simulink model "ECB"  (R2017a)
settings: Solver=ode4  StartTime=0.0  StopTime=1548.3  FixedStep=0.001  RelTol=1e-3  EnableMultiTasking=on
undefined symbols (not defined in the file or in its folder): magnitude, sgn, sigbuilder_block
libraries: simulink x1
(part 2 of 2)

== system ECB/ECB Model/Driver, Ctrl & Motor/AC-motor/Voltage Equations ==
  us : Inport
  is : Inport  Port=2
  wM : Inport  Port=3
  Gain1 : Gain  Gain=1i*p
  Gain2 : Gain  Gain=Rs
  Integrator (Complex Signal) : Subsystem
      mask Display: disp('1/s');
  Product : Product
  Sum1 : Sum  Inputs=+--
  psis : Outport
  wires:
  wM/1 -> Gain1/1
  Integrator (Complex Signal)/1(y) -> psis/1, Product/2
  Sum1/1 -> Integrator (Complex Signal)/1(u)
  us/1 -> Sum1/1
  Gain1/1 -> Product/1
  Product/1 -> Sum1/3
  is/1 -> Gain2/1
  Gain2/1 -> Sum1/2

== system ECB/ECB Model/Driver, Ctrl & Motor/Driver/Cycle ==
  Demux : Demux  Tag=STV Demux  Outputs=1
  FromWs : FromWorkspace  Tag=STV FromWs  VariableName=tuvar  SampleTime=0  OutputAfterFinalValue=Setting to zero
      SigBuilderData=|
      | common.afterFinalStr = 'Set to zero'
      | common.sampleTime = '0'
      | dataSet(1).timeRange = [0 1548.3]
      | dataSet(1).name = 'E11_TFBest'
      | dataSet(2).timeRange = [0 1767.7]
      | dataSet(2).name = 'Brauschweig'
      | dataSet(3).timeRange = [0 1548.3]
      | dataSet(3).name = 'NYbus'
      | dataSet(4).timeRange = [0 1698.1]
      | dataSet(4).name = 'ft5v'
      | dataSet(5).timeRange = [0 1548.3]
      | dataSet(5).name = 'ft9v'
      | dataSet(6).timeRange = [0 1548.3]
      | dataSet(6).name = 'ft11v'
      | dataSet(7).timeRange = [0 1549.6]
      | dataSet(7).name = 'ft19v'
      | dataSet(8).timeRange = [0 1798.1]
      | dataSet(8).name = 'ft25v'
      | dataSet(9).timeRange = [0 2058.9]
      | dataSet(9).name = 'tf4v'
      | dataSet(10).timeRange = [0 1565.4]
      | dataSet(10).name = 'tf8v'
      | dataSet(11).timeRange = [0 1548.3]
      | dataSet(11).name = 'tf12v'
      | dataSet(12).timeRange = [0 1569]
      | dataSet(12).name = 'tf22v'
      | dataSet(13).timeRange = [0 1548.3]
      | dataSet(13).name = 'tf24v'
      | sbobj.Name = 'Signal Builder'
      | sbobj.Groups(1).Name = 'E11_TFBest'
      | sbobj.Groups(1).Signals.Name = 'vel'
      | sbobj.Groups(1).Signals.XData = [0 0.1 0.2 0.3 0.4 0.5 0.6 0.7 0.8 0.9 1 1.1 ... (15484 elements, 1x15484)]
      | sbobj.Groups(1).Signals.YData = [0 0 0 0 0 0 0 0 0 0 0 0 ... (15484 elements, 1x15484)]
      | sbobj.Groups(1).TimeRange = [0 1548.3]
      | sbobj.Groups(2).Name = 'Brauschweig'
      | sbobj.Groups(2).Signals.Name = 'vel'
      | sbobj.Groups(2).Signals.XData = [0 0.09 0.2 0.3 0.39 0.5 0.59 0.7 0.8 0.89 1 1.09 ... (17678 elements, 1x17678)]
      | sbobj.Groups(2).Signals.YData = [1.0444e-14 1.3228e-14 1.6325e-14 1.9741e-14 2.3481e-14 2.7541e-14 3.1914e-14 3.6586e-14 4.1533e-14 4.6723e-14 5.2115e-14 5.7653e-14 ... (17678 elements, 1x17678)]
      | sbobj.Groups(2).TimeRange = [0 1767.7]
      | sbobj.Groups(3).Name = 'NYbus'
      | sbobj.Groups(3).Signals.Name = 'vel'
      | sbobj.Groups(3).Signals.XData = [0 14.4398340249 15.569428651 16.6194998155 17.1824897772 18.2271388874 20.195344564 22.1671649434 24.6947458789 24.7290855555 25.2468917321 27.1554548124 27.5377096339 27.9922585115 29.4571168227 29.9134730516 31.3692946058 59.7510373444 60.2814949808 61.438199878 62.5714092069 62.6418959116 63.6666641565 64.6769735901 67.1159943068 70.1631887703 73.0892906899 75.1352124767 76.7844206309 78.4209773253 78.9839672869 79.0255363692 80.5446152224 82.9800212364 84.4231913307 86.488993983 88.8864456175 89.7991580755 91.1555753025 92.4794602044 94.3609130137 95.6956420239 97.5933609959 163.815620034 165.336506239 165.977212311 168.109886965 171.063099156 171.887251395 174.273858921 209.128630705 211.228773034 212.935816433 214.5 216.99332033 220.020633929 221.936426414 223.32899067 225.194177316 225.243571477 226.617466545 227.55186722 232.033195021 233.595650308 234.147796161 234.758311934 235.304501058 236.762129964 237.184146516 240.133744004 243.240581063 246.154031523 247.063129278 248.962655602 284.813278008 287.056201098 288.723482766 291.678502308 294.718467366 297.409613603 300.248962656 330.124481328 331.808029159 332.961119353 334.067218411 337.485823587 340.536632754 343.935357065 344.822766603 346.208101453 346.637347411 350.041493776 389.377593361 391.017764758 391.618709099 394.157134143 398.586048753 400.641007297 402.192618476 404.065034528 405.416029701 407.302904564 434.68879668 435.789473684 436.910031553 438.4851383 441.858559692 442.242621864 445.147035567 479.502074689 481.133209329 482.298950983 484.368368338 486.332959312 488.402376667 491.85532152 494.991076202 496.96108923 499.486862814 502.907275342 504.269114624 506.108998351 507.470837632 510.373443983 555.186721992 556.347041592 557.932992447 557.983598286 562.425164356 565.506698496 568.311707872 569.697042721 572.614107884 1548.3]
      | sbobj.Groups(3).Signals.YData = [0 0 7.56479303085 10.6316010163 14.3117705989 17.0718977858 15.7429476588 14.6184513975 16.7652169873 18.7075287114 19.8320249728 15.1295860617 8.58706235935 6.13361597096 4.49798504537 2.14676558984 0 0 1.84008479129 10.9382818149 18.7075287114 22.6943790926 24.3300100181 25.1478254809 22.2854713612 25.6589601452 22.1832444283 25.2500524138 34.0415686388 42.1174963339 45.7976659165 48.1488853721 49.5800624319 46.5132544465 43.6509003267 47.8422045735 42.6286309982 37.9261920871 30.1569451906 20.5476135027 14.3117705989 5.31580050817 0 0 1.43117705989 9.50710475499 17.4808055172 15.5384937931 5.82693517241 0 0 6.13361597096 18.1963940472 23.5 22.387698294 24.6366908167 20.343159637 14.6184513975 7.462566098 4.60021197822 3.47571571688 0 0 3.88462344828 6.95143143376 13.0850474047 16.0496284574 14.0050898004 9.71155862069 7.56479303085 14.3117705989 10.1204663521 5.21357357532 0 0 14.2095436661 24.0233292196 22.1832444283 25.1478254809 8.38260849365 0 0 10.7338279492 19.6275711071 25.8634140109 22.0810174955 25.6589601452 20.7520673684 14.6184513975 8.4848354265 4.60021197822 0 0 8.2803815608 14.1073167332 16.8674439201 13.9028628675 17.4808055172 20.7520673684 14.0050898004 5.92916210526 0 0 5.92916210526 12.9828204719 17.5830324501 11.2449626134 4.80466584392 0 0 7.76924689655 17.3785785844 21.7743366969 20.2409327042 24.6366908167 22.7966060254 31.1792145191 29.9524913249 31.9970299819 28.3168603993 20.8542943013 12.2672319419 4.80466584392 0 0 9.30265088929 14.5162244646 17.3785785844 15.1295860617 20.4453865699 10.1204663521 3.98685038113 0 0]
      | sbobj.Groups(3).TimeRange = [0 1548.3]
      | sbobj.Groups(4).Name = 'ft5v'
      | sbobj.Groups(4).Signals.Name = 'vel'
      | sbobj.Groups(4).Signals.XData = [0 0.1 0.2 0.3 0.4 0.5 0.6 0.7 0.8 0.9 1 1.1 ... (16982 elements, 1x16982)]
      | sbobj.Groups(4).Signals.YData = [3.68548 3.78425333333 3.859568 4.08498285714 4.35425777778 4.58117454545 4.78955692308 5.01645066667 5.233752 5.448584 5.66218133333 5.922696 ... (16982 elements, 1x16982)]
      | sbobj.Groups(4).TimeRange = [0 1698.1]
      | sbobj.Groups(5).Name = 'ft9v'
      | sbobj.Groups(5).Signals.Name = 'vel'
      | sbobj.Groups(5).Signals.XData = [0 0.1 0.2 0.3 0.4 0.5 0.6 0.7 0.8 0.9 1 1.1 ... (14571 elements, 1x14571)]
      | sbobj.Groups(5).Signals.YData = [4.57444 4.92014666667 5.318944 5.75442857143 6.18568 6.59480363636 7.04329846154 7.48701866667 7.90557066667 8.34017333333 8.75996 9.17974666667 ... (14571 elements, 1x14571)]
      | sbobj.Groups(5).TimeRange = [0 1548.3]
      | sbobj.Groups(6).Name = 'ft11v'
      | sbobj.Groups(6).Signals.Name = 'vel'
      | sbobj.Groups(6).Signals.XData = [0 0.1 0.2 0.3 0.4 0.5 0.6 0.7 0.8 0.9 1 1.1 ... (13984 elements, 1x13984)]
      | sbobj.Groups(6).Signals.YData = [1.27788 1.33344 1.46308 1.53980571429 1.66268444444 1.76613454545 1.87906769231 1.99892533333 2.11004533333 2.21005333333 2.31746933333 2.42118133333 ... (13984 elements, 1x13984)]
      | sbobj.Groups(6).TimeRange = [0 1548.3]
      | sbobj.Groups(7).Name = 'ft19v'
      | sbobj.Groups(7).Signals.Name = 'vel'
      | sbobj.Groups(7).Signals.XData = [0 0.1 0.2 0.3 0.4 0.5 0.6 0.7 0.8 0.9 1 1.1 ... (15497 elements, 1x15497)]
      | sbobj.Groups(7).Signals.YData = [3.8892 4.21021333333 4.544808 4.92102857143 5.34610666667 5.71931272727 6.08168307692 6.378288 6.69806666667 6.993152 7.29194133333 7.58826133333 ... (15497 elements, 1x15497)]
      | sbobj.Groups(7).TimeRange = [0 1549.6]
      | sbobj.Groups(8).Name = 'ft25v'
      | sbobj.Groups(8).Signals.Name = 'vel'
      | sbobj.Groups(8).Signals.XData = [0 0.1 0.2 0.3 0.4 0.5 0.6 0.7 0.8 0.9 1 1.1 ... (17982 elements, 1x17982)]
      | sbobj.Groups(8).Signals.YData = [4.92632 5.43870666667 5.752312 6.23330285714 6.68777777778 7.04433454545 7.40515076923 7.752472 8.10682133333 8.42166133333 8.71304266667 9.02417866667 ... (17982 elements, 1x17982)]
      | sbobj.Groups(8).TimeRange = [0 1798.1]
      | sbobj.Groups(9).Name = 'tf4v'
      | sbobj.Groups(9).Signals.Name = 'vel'
      | sbobj.Groups(9).Signals.XData = [0 0.1 0.2 0.3 0.4 0.5 0.6 0.7 0.8 0.9 1 1.1 ... (20590 elements, 1x20590)]
      | sbobj.Groups(9).Signals.YData = [2.53724 2.86442666667 3.174328 3.52144571429 3.72252 3.88751636364 4.10146769231 4.374424 4.64605066667 4.90533066667 5.17201866667 5.45352266667 ... (20590 elements, 1x20590)]
      | sbobj.Groups(9).TimeRange = [0 2058.9]
      | sbobj.Groups(10).Name = 'tf8v'
      | sbobj.Groups(10).Signals.Name = 'vel'
      | sbobj.Groups(10).Signals.XData = [0 0.1 0.2 0.3 0.4 0.5 0.6 0.7 0.8 0.9 1 1.1 ... (15655 elements, 1x15655)]
      | sbobj.Groups(10).Signals.YData = [0 0 0 0 0 0 0 0 0 0 0 0 ... (15655 elements, 1x15655)]
      | sbobj.Groups(10).TimeRange = [0 1565.4]
      | sbobj.Groups(11).Name = 'tf12v'
      | sbobj.Groups(11).Signals.Name = 'vel'
      | sbobj.Groups(11).Signals.XData = [0 0.1 0.2 0.3 0.4 0.5 0.6 0.7 0.8 0.9 1 1.1 ... (14670 elements, 1x14670)]
      | sbobj.Groups(11).Signals.YData = [5.05596 5.07448 5.193008 5.51896 5.82145333333 6.13517090909 6.42216615385 6.73881066667 7.026488 7.33638933333 7.66110666667 7.99446666667 ... (14670 elements, 1x14670)]
      | sbobj.Groups(11).TimeRange = [0 1548.3]
      | sbobj.Groups(12).Name = 'tf22v'
      | sbobj.Groups(12).Signals.Name = 'vel'
      | sbobj.Groups(12).Signals.XData = [0 0.1 0.2 0.3 0.4 0.5 0.6 0.7 0.8 0.9 1 1.1 ... (15691 elements, 1x15691)]
      | sbobj.Groups(12).Signals.YData = [15.53828 14.3962133333 14.22336 14.1783828571 14.4414844444 14.6038618182 14.8444923077 15.0962693333 15.182696 15.4185173333 15.664216 15.9259653333 ... (15691 elements, 1x15691)]
      | sbobj.Groups(12).TimeRange = [0 1569]
      | sbobj.Groups(13).Name = 'tf24v'
      | sbobj.Groups(13).Signals.Name = 'vel'
      | sbobj.Groups(13).Signals.XData = [0 0.1 0.2 0.3 0.4 0.5 0.6 0.7 0.8 0.9 1 1.1 ... (15122 elements, 1x15122)]
      | sbobj.Groups(13).Signals.YData = [2.4076 2.48168 2.489088 2.51342857143 2.58868444444 2.69718545455 2.81361538462 2.92739466667 3.03481066667 3.144696 3.241 3.366936 ... (15122 elements, 1x15122)]
      | sbobj.Groups(13).TimeRange = [0 1548.3]
  vel : Outport  Tag=STV Outport
  wires:
  Demux/1 -> vel/1
  FromWs/1 -> Demux/1

== system ECB/ECB Model/Driver, Ctrl & Motor/Driver/Signal Builder ==
  Demux : Demux  Tag=STV Demux  Outputs=1
  FromWs : FromWorkspace  Tag=STV FromWs  VariableName=tuvar  SampleTime=0
      SigBuilderData=|
      | common.afterFinalStr = 'Extrapolate'
      | common.sampleTime = 0
      | dataSet.timeRange = [0 60]
      | dataSet.name = 'Group 1'
      | sbobj.Groups.Name = 'Group 1'
      | sbobj.Groups.Signals.Name = 'Signal 1'
      | sbobj.Groups.Signals.XData = [0 5 20 35 55 60]
      | sbobj.Groups.Signals.YData = [0 0 60 60 0 0]
      | sbobj.Groups.TimeRange = [0 60]
  Signal 1 : Outport  Tag=STV Outport
  wires:
  Demux/1 -> Signal 1/1
  FromWs/1 -> Demux/1

== system ECB/ECB Model/Driver, Ctrl & Motor/PID Current Ctrl/Derivative (Complex Signla) ==
  x : Inport
  Complex to Real-Imag : ComplexToRealImag
  Derivative : Derivative
  Derivative1 : Derivative
  Real-Imag to Complex : RealImagToComplex
  dx : Outport
  wires:
  Complex to Real-Imag/2 -> Derivative1/1
  Real-Imag to Complex/1 -> dx/1
  Derivative1/1 -> Real-Imag to Complex/2
  x/1 -> Complex to Real-Imag/1
  Derivative/1 -> Real-Imag to Complex/1
  Complex to Real-Imag/1 -> Derivative/1

== system ECB/ECB Model/Driver, Ctrl & Motor/PID Current Ctrl/Integrator (Complex Signal) ==
  u : Inport
  Complex to Real-Imag : ComplexToRealImag
  Integrator : Integrator
  Integrator1 : Integrator
  Real-Imag to Complex : RealImagToComplex
  y : Outport
  wires:
  u/1 -> Complex to Real-Imag/1
  Real-Imag to Complex/1 -> y/1
  Integrator1/1 -> Real-Imag to Complex/2
  Integrator/1 -> Real-Imag to Complex/1
  Complex to Real-Imag/2 -> Integrator1/1
  Complex to Real-Imag/1 -> Integrator/1

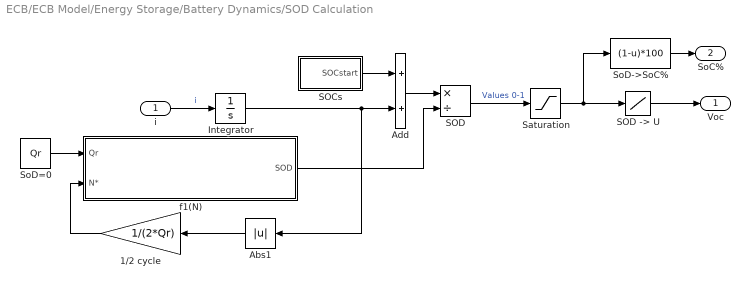
== system ECB/ECB Model/Energy Storage/Battery Dynamics/SOD Calculation ==
  i : Inport
  1/2 cycle : Gain  Gain=1/(2*Qr)
  Abs1 : Abs
  Add : Sum
  Integrator : Integrator
  SOCs : Subsystem
  SOD : Product  Inputs=*/
  "SOD -> U" : Lookup_n-D  NumberOfTableDimensions=1  BreakpointsForDimension1=SOD  BreakpointsForDimension2=[4.2,2.5]  BreakpointsForDimension3=[5, 7]  Table=VOLT  InternalRulePriority=Speed  RndMeth=Simplest  InputSameDT=on
  Saturation : Saturate  UpperLimit=1  LowerLimit=0
  SoD->SoC% : Fcn  Expr=(1-u)*100
  SoD=0 : Constant  Value=Qr
  f1(N) : Subsystem
  Voc : Outport
  SoC% : Outport  Port=2
  wires:
  SOD/1 -> Saturation/1  "Values 0-1"
  SoD=0/1 -> f1(N)/1(Qr)
  1/2 cycle/1 -> f1(N)/2(N*)
  "SOD -> U"/1 -> Voc/1
  Abs1/1 -> 1/2 cycle/1
  Add/1 -> SOD/1
  i/1 -> Integrator/1  "i"
  SoD->SoC%/1 -> SoC%/1
  f1(N)/1(SOD) -> SOD/2
  Saturation/1 -> SoD->SoC%/1, "SOD -> U"/1
  SOCs/1(SOCstart) -> Add/1
  Integrator/1 -> Add/2, Abs1/1

== system ECB/ECB Model/Driver, Ctrl & Motor/AC-motor/Voltage Equations/Integrator (Complex Signal) ==
  u : Inport
  Complex to Real-Imag : ComplexToRealImag
  Integrator : Integrator
  Integrator1 : Integrator
  Real-Imag to Complex : RealImagToComplex
  y : Outport
  wires:
  u/1 -> Complex to Real-Imag/1
  Real-Imag to Complex/1 -> y/1
  Integrator1/1 -> Real-Imag to Complex/2
  Integrator/1 -> Real-Imag to Complex/1
  Complex to Real-Imag/2 -> Integrator1/1
  Complex to Real-Imag/1 -> Integrator/1

== system ECB/ECB Model/Energy Storage/Battery Dynamics/SOD Calculation/SOCs ==
  SOC0 : Gain  Gain=1-(SOC0/100)
  Soc=? : Constant  Value=Qr
  SOCstart : Outport
  wires:
  SOC0/1 -> SOCstart/1
  Soc=?/1 -> SOC0/1

== system ECB/ECB Model/Energy Storage/Battery Dynamics/SOD Calculation/f1(N) ==
  Qr : Inport
  N* : Inport  Port=2
  N+N* : Sum
  N+N*1 : Sum  Inputs=+-
  N0 : Constant  Value=N0
  Product1 : Product
  f1(N)1 : Gain  Gain=0.2/Nnom
  SOD : Outport
  wires:
  Qr/1 -> N+N*1/1, f1(N)1/1
  Product1/1 -> N+N*1/2
  f1(N)1/1 -> Product1/1
  N+N*/1 -> Product1/2
  N0/1 -> N+N*/1
  N*/1 -> N+N*/2
  N+N*1/1 -> SOD/1

== matlab function ECB/ECB Model/Driver, Ctrl & Motor/PID Current Ctrl/MATLAB Function ==
  data: usref input; usref_saturated output; Umax input; usref_limit output
function [usref_saturated, usref_limit] = fcn(usref, Umax)
%#codegen

im1 = imag(usref);
re1 = real(usref);
alpha = atan2(im1,re1);

uref = sqrt(im1^2+re1^2);

if uref > (2/3)*Umax
    
    im2 = (2/3)*Umax*sin(alpha);
    re2 = (2/3)*Umax*cos(alpha);
    usref_saturated = re2+1i*im2;
    
else
    
    usref_saturated = usref;
    
end

usref_limit = sqrt(((2/3)*Umax*sin(alpha))^2+((2/3)*Umax*cos(alpha))^2);

== matlab function ECB/ECB Model/Driver, Ctrl & Motor/Regenerative Braking and Current Limits/MATLAB Function ==
  data: isref input; is_limited output; Ich_m input; soc input; brakes output; Ids_max output; Ich_max output; soclim input; v input; vlimPartial input; a input; alimPartial input; Ids_m input; Ubat input; Umax input; mode output
function [is_limited, brakes, Ids_max, Ich_max, mode] = fcn(isref, Ich_m, soc, soclim, v,...
    vlimPartial, a, alimPartial, Ids_m, Ubat, Umax)
% This function handles the regenerative braking algorithm. 
% The algorithm also ensures that the current does not exceed the limits.
% Furthermore, the current is limited during regenerative braking such that the battery voltage does not exceed its limits.

% There are 2 types of breaking modes:

% 1. Regeneration disabled
%   - if SOC above threshold (def 90%) 
%   - OR if deceleration more than threshold (def 4 m/s^2)
%   - OR if speed is less than threshold (def 4 km/h)
% 2. Regeneration enabled
%   - if SOC below threshold (def 90%) %
%   - AND if deceleration below threshold (def 4 m/s^2)
%   - AND if speed is more than threshold (def 4 km/h)

threshold_voltage = 0.92;

iq = imag(isref);  %id is zero and so is=iq has only an imaginary value.

Ids_max = Ids_m; % [A] Maximum current the motor can handle when in motoring mode.
Ich_max = Ich_m; % [A] Maximum current the motor can handle when in regeneration mode.

brakes = 0; %by default, brakes are not used
is_limited=1i*iq;
%mode=0; %motoring

if iq >= 0 %|| v > 50
%0. MOTORING
    if abs(iq) > Ids_max %If reference current is larger than the limit, then saturate
        is_limited=1i*Ids_max;
        mode=0; %motoring
    else
        is_limited=1i*iq;
        mode=0; %motoring
    end

%BRAKING/REGENERATION
else

    %2. REGENERATION ENABLED
    if soc < soclim && a < alimPartial && v > vlimPartial
    % Deceleration has to be less than limit AND speed more than limit.
    brakes=1; % Using brakes
    mode=2; % Regeneration enabled
        if v >= vlimPartial+1
            if iq > -Ich_max % Saturating charging current to the limit
                is_limited=1i*iq;
            else
                is_limited=-1i*Ich_max;
            end
        elseif v < vlimPartial+1 && v > vlimPartial % Make a smooth transition to using mechanical brakes only.
            if iq > -Ich_max % Saturating charging current to the limit
                is_limited=(v-vlimPartial)*1i*iq;
            else
                is_limited=(v-vlimPartial)*(-1i*Ich_max);
            end
        end

    %1. REGENERATION DISABLED
    else
    % First, decide if we want to use regenerative braking at all,
    % depending on the battery SOC level, deceleration and speed.
    brakes=1; % Using brakes
    mode=1; % No reg.
    is_limited=1i*0; % No regeneration is allowed.
    end
    
    % LIMITING CHARGING CURRENT IF VOLTAGE GETS TOO HIGH
    if Ubat > threshold_voltage*Umax
        is_limited=1i*min(imag(is_limited)*((Umax-Ubat)/(Umax*(1-threshold_voltage)))^(1),0);
    end
        
end

end

== matlab function ECB/ECB Model/Driver, Ctrl & Motor/PID Speed Ctrl/MATLAB Function: Amplify kps if wM_ref == 0 ==
  data: wM_ref input; kps input; kps2 output; multiplier input
function kps2 = fcn(wM_ref,kps, multiplier)

if wM_ref == 0
    kps2 = multiplier*kps;
else
    kps2 = kps;
end

== matlab function ECB/ECB Model/Driver, Ctrl & Motor/Field Weakening/MATLAB Function ==
  data: is_limited input; is_ref output; Ubat input; wM input; p input; i input; tRout input; flux input; Ls input; Ich input; Ids input; Rs input
function is_ref = fcn(is_limited,Ubat,wM,p,i,tRout,flux,Ls,Ich,Ids,Rs)

speed_kmh = wM/i*tRout*3.6;
is_limited_orig = 1i*is_limited;
if is_limited >= 0
    Imax = Ids;
else
    Imax = Ich;
end
w_m = p*wM;
umax = (2/3)*Ubat;
c_resolution = 0.1;

fw_threshold = 10; % !!! (km/h)The minimum speed for field-weakening to be deployed !!!

if speed_kmh > fw_threshold
    % Implement field-weakening here
    if sqrt((-1*w_m*Ls*is_limited)^2+(Rs*is_limited+w_m*flux)^2) > umax
        % Implement field-weakening here
        
        c = -c_resolution;
        j = 0;
        
        while j == 0
            if sqrt(complex((Rs*c-w_m*Ls*is_limited)^2+(Rs*is_limited+w_m*Ls*c+w_m*flux)^2)) <= umax || abs(c) >= Imax
                j = 1;
            else
                c = c - c_resolution;
            end
        end
        
        new_id = c - c_resolution;
        is_ref = new_id + 1i*is_limited;

        if abs(is_ref) > Imax
            % Calculate new idref and iqref here
            c = -c_resolution;
            j = 0;
            while j == 0
                iq_temp = sqrt(complex(Imax^2-c^2));
                
                if sqrt(complex((Rs*c-w_m*Ls*iq_temp)^2+(Rs*iq_temp+w_m*Ls*c+w_m*flux)^2)) <= umax || abs(c) >= Imax
                    j = 1;
                else
                    c = c - c_resolution;
                end
            end
            new_id = c - c_resolution;
            new_iq = sign(is_limited)*sqrt(complex(Imax^2-(c-c_resolution)^2));
            is_ref = new_id + 1i*new_iq;
        end
    else
        is_ref = 0+is_limited_orig;
    end
else
    is_ref = 0+is_limited_orig;
end
